simulink model "PID_Pendule"  (R2025a)
settings: Solver=VariableStepAuto  StartTime=0.0  StopTime=10  RelTol=1e-3
values from neighbouring files (symbols this model uses):
  f = 1e-3    (= 0.001)    [pendule2.m]
  g = 9.81    [pendule2.m]
  Kd = 0.5    [pendule2.m]
  Ki = 20    [pendule2.m]
  Kp = 10    [pendule2.m]
  l = 0.3    [pendule2.m]
  m = 0.5    [pendule2.m]
  omega_0 = 0    [pendule2.m]
  theta_0 = pi/6    (= 0.523598775598)    [pendule2.m]
  theta_r = pi/3    (= 1.0471975512)    [pendule2.m]
undefined symbols (not defined in the file or in its folder): F, G
libraries: simulink x1
settings Model: Creator=vikfo  LastModifiedBy=vikfo

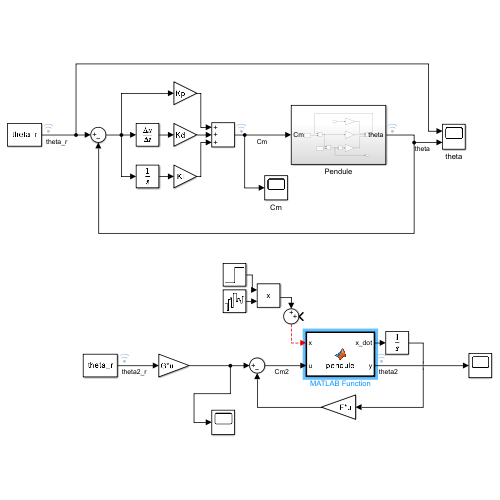
[thumbnail: Simulink's stored preview of the top-level diagram]
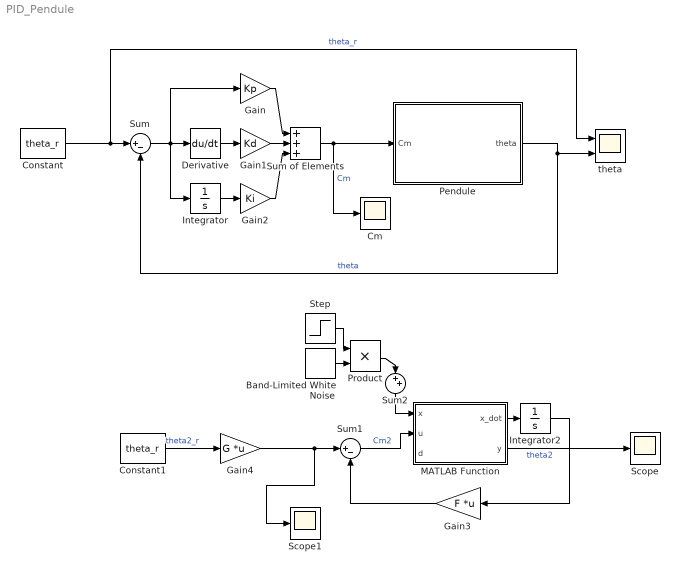
== system PID_Pendule ==
  Band-Limited White Noise : simulink/Sources/Band-Limited White Noise  Cov=[0.01]  Ts=0.1  seed=[23341]
  Cm : Scope
      settings: ActiveDisplayYMinimum=-6.7398599898829827  ActiveDisplayYMaximum=7.1977650122094543
  Constant : Constant  Value=theta_r
  Constant1 : Constant  Value=theta_r
  Derivative : Derivative
  Gain : Gain  Gain=Kp
  Gain1 : Gain  Gain=Kd
  Gain2 : Gain  Gain=Ki
  Gain3 : Gain  Gain=F  Multiplication=Matrix(K*u)
  Gain4 : Gain  Gain=G  Multiplication=Matrix(K*u)
  Integrator : Integrator
  Integrator2 : Integrator  InitialCondition=[theta_0 omega_0]
  MATLAB Function : MATLAB Function  TreatAsAtomicUnit=on
  Pendule : Subsystem
  Product : Product
  Scope : Scope
      settings: ActiveDisplayYMinimum=-1  ActiveDisplayYMaximum=1  DataLoggingVariableName=ScopeData2
  Scope1 : Scope
      settings: DataLoggingVariableName=ScopeData3
  Step : Step  Time=6  SampleTime=0
  Sum : Sum  Inputs=|+-
  Sum of Elements : Sum  Inputs=+++
  Sum1 : Sum  Inputs=|+-
  Sum2 : Sum  Inputs=|++
  theta : Scope  NumInputPorts=2
      settings: ActiveDisplayYMinimum=0.42158126344051738  ActiveDisplayYMaximum=1.4417563850183324
  wires:
  Pendule/1(theta) -> theta/2, Sum/2  "theta"
  Constant/1 -> theta/1, Sum/1  "theta_r"
  Sum/1 -> Derivative/1, Integrator/1, Gain/1
  Derivative/1 -> Gain1/1
  Integrator/1 -> Gain2/1
  Gain1/1 -> Sum of Elements/2
  Sum of Elements/1 -> Cm/1, Pendule/1(Cm)  "Cm"
  Gain/1 -> Sum of Elements/1
  Gain2/1 -> Sum of Elements/3
  Constant1/1 -> Gain4/1  "theta2_r"
  Sum1/1 -> MATLAB Function/2(u)  "Cm2"
  MATLAB Function/1(x_dot) -> Integrator2/1
  Integrator2/1 -> Gain3/1
  Gain3/1 -> Sum1/2
  Gain4/1 -> Scope1/1, Sum1/1
  MATLAB Function/2(y) -> Scope/1  "theta2"
  Sum2/1 -> MATLAB Function/1(x)
  Product/1 -> Sum2/1
  Step/1 -> Product/1
  Band-Limited White Noise/1 -> Product/2

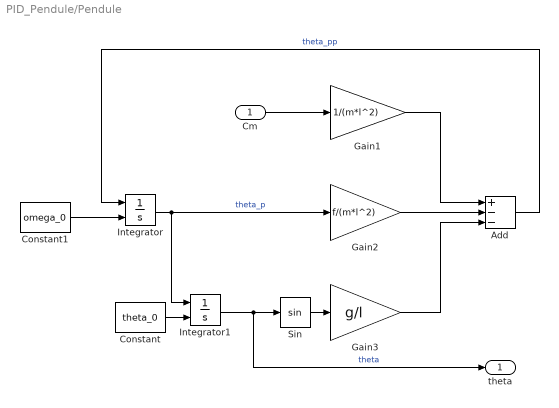
== system PID_Pendule/Pendule ==
  Cm : Inport
  Add : Sum  Inputs=+--
  Constant : Constant  Value=theta_0
  Constant1 : Constant  Value=omega_0
  Gain1 : Gain  Gain=1/(m*l^2)
  Gain2 : Gain  Gain=f/(m*l^2)
  Gain3 : Gain  Gain=g/l
  Integrator : Integrator  InitialConditionSource=external
  Integrator1 : Integrator  InitialConditionSource=external
  Sin : Trigonometry
  theta : Outport
  wires:
  Gain2/1 -> Add/2
  Integrator1/1 -> theta/1, Sin/1  "theta"
  Integrator/1 -> Integrator1/1, Gain2/1  "theta_p"
  Gain3/1 -> Add/3
  Cm/1 -> Gain1/1
  Add/1 -> Integrator/1  "theta_pp"
  Gain1/1 -> Add/1
  Sin/1 -> Gain3/1
  Constant/1 -> Integrator1/2
  Constant1/1 -> Integrator/2

== matlab function PID_Pendule/MATLAB Function ==
  data: x input; x_dot output; u input; y output; d input
function [x_dot, y]= pendule(x, u,d)


g = 9.81;  

% Masse du pendule (kg)
m = 0.5;  
% Longueur du pendule (m)
l = 0.3;

% Coefficient de frottement fluide (N.m.s/rad)
f = 1e-3;

A =[0 1;
    -g/l 0];

B = [0;
     1];

C = [1 0];

E = [1 0];

x_dot = A*x + B*u +E*d;
y = C*x;

%x_dot[0] = x[1]
%x_dot[1] = -f/(m*l^2) * x[1] - x[0] + Cm/(m*l^2)
%x_dot[2] = x[0]
